simulink model "sf_abstemporal_ct"  (Simulink 7.6)
settings: Solver=VariableStepDiscrete  StartTime=0.0  StopTime=10.0  MaxStep=.2  RelTol=1e-3
settings Model: Creator=The MathWorks Inc.
settings DebuggingCC: StrictBusMsg=Warning
settings SFSimCC: SimParseCustomCode=off

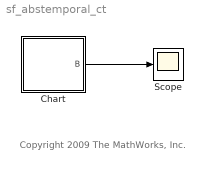
== system sf_abstemporal_ct ==
  note: Copyright 2009 The MathWorks, Inc.
  Chart : Stateflow chart  TreatAsAtomicUnit=on
  Scope : Scope
  wires:
  Chart/1(B) -> Scope/1

== stateflow chart Chart ==
  settings: updateMethod=CONTINUOUS
  state A
  state B
  (default) -> A
  A -> B : after(4.2345, sec)
  data: B output boolean
